simulink model "pv_array"  (R2015a)
settings: Solver=ode45  StartTime=0.0  StopTime=10.0  RelTol=1e-3
libraries: powerlib x4
settings Model: Creator=Limon  LastModifiedBy=Limon

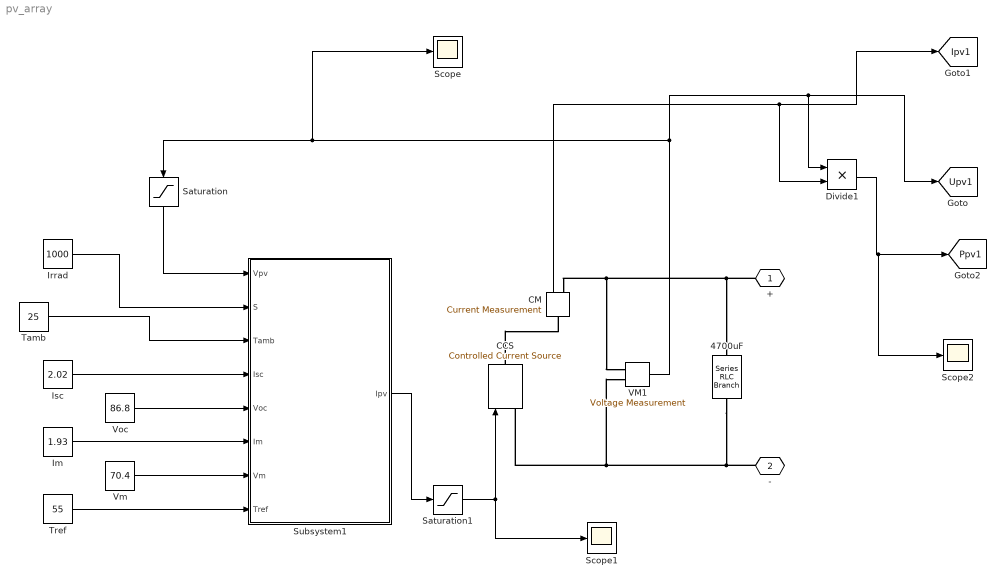
== system pv_array ==
  4700uF : powerlib/Elements/Series RLC Branch  LConnTagsString=__new0  RConnTagsString=__new0  BranchType=C  Resistance=1  Inductance=5e-03  SetiL0=off  InitialCurrent=0  Capacitance=4700e-6  Setx0=off  InitialVoltage=0  Measurements=None
  CCS : powerlib/Electrical Sources/Controlled Current Source  Initialize=on  Source_Type=AC  Amplitude=0  Phase=0  Frequency=0  Measurements=None
  CM : powerlib/Measurements/Current Measurement  PhasorSimulation=off  OutputType=Complex  PSBequivalent=0
  Divide1 : Product  Inputs=**
  Im : Constant  Value=1.93
  "Irrad " : Constant  Value=1000
  Isc : Constant  Value=2.02
  Saturation : Saturate  UpperLimit=100  LowerLimit=0
  Saturation1 : Saturate  UpperLimit=4  LowerLimit=0
  Scope : Scope
  Scope1 : Scope
  Scope2 : Scope
      settings: SaveName=ScopeData2
  Subsystem1 : Subsystem
  "Tamb " : Constant  Value=25
  Tref : Constant  Value=55
  VM1 : powerlib/Measurements/Voltage Measurement  PhasorSimulation=off  OutputType=Complex  PSBequivalent=0
  Vm : Constant  Value=70.4
  Voc : Constant  Value=86.8
  + : PMIOPort  Tag=PMCPort  Port=1  Side=Left
  - : PMIOPort  Tag=PMCPort  Port=2  Side=Right
  tag scope: Ipv1=global, Ppv1=global, Upv1=global
  wires:
  Saturation1/1 -> CCS/1, Scope1/1
  CM/1 -> Divide1/2, [Ipv1]
  Divide1/1 -> Scope2/1, [Ppv1]
  Subsystem1/1(Ipv) -> Saturation1/1
  Tref/1 -> Subsystem1/8(Tref)
  VM1/1 -> Divide1/1, [Upv1], Scope/1, Saturation/1
  Saturation/1 -> Subsystem1/1(Vpv)
  Vm/1 -> Subsystem1/7(Vm)
  Voc/1 -> Subsystem1/5(Voc)
  Im/1 -> Subsystem1/6(Im)
  Isc/1 -> Subsystem1/4(Isc)
  "Tamb "/1 -> Subsystem1/3(Tamb)
  "Irrad "/1 -> Subsystem1/2(S)
  connections:
  -/RConn1 -- 4700uF/RConn1 -- VM1/LConn2 -- CCS/LConn1
  +/RConn1 -- 4700uF/LConn1 -- VM1/LConn1 -- CM/RConn1
  CCS/RConn1 -- CM/LConn1

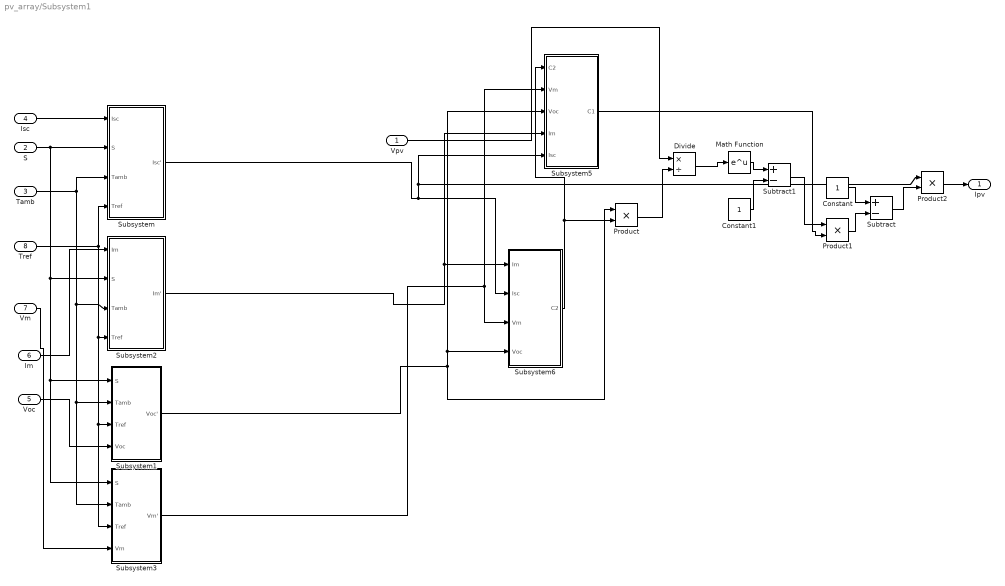
== system pv_array/Subsystem1 ==
  Vpv : Inport
  S : Inport  Port=2
  Tamb : Inport  Port=3
  Isc : Inport  Port=4
  Voc : Inport  Port=5
  Im : Inport  Port=6
  Vm : Inport  Port=7
  Tref : Inport  Port=8
  Constant : Constant
  Constant1 : Constant
  Divide : Product  Inputs=*/
  Math Function : Math  SaturateOnIntegerOverflow=on
  Product : Product  RndMeth=Zero
  Product1 : Product  RndMeth=Zero
  Product2 : Product  RndMeth=Zero
  Subsystem : Subsystem
  Subsystem1 : Subsystem
  Subsystem2 : Subsystem
  Subsystem3 : Subsystem
  Subsystem5 : Subsystem
  Subsystem6 : Subsystem
  Subtract : Sum  Inputs=+-
  Subtract1 : Sum  Inputs=+-
  Ipv : Outport
  wires:
  Vm/1 -> Subsystem3/4(Vm)
  Voc/1 -> Subsystem1/4(Voc)
  Im/1 -> Subsystem2/1(Im)
  Tref/1 -> Subsystem/4(Tref), Subsystem2/4(Tref), Subsystem3/3(Tref), Subsystem1/3(Tref)
  Tamb/1 -> Subsystem/3(Tamb), Subsystem2/3(Tamb), Subsystem3/2(Tamb), Subsystem1/2(Tamb)
  S/1 -> Subsystem/2(S), Subsystem2/2(S), Subsystem3/1(S), Subsystem1/1(S)
  Isc/1 -> Subsystem/1(Isc)
  Subsystem5/1(C1) -> Product1/2
  Vpv/1 -> Divide/1
  Subsystem6/1(C2) -> Product/2, Subsystem5/1(C2)
  Subsystem3/1(Vm') -> Subsystem6/3(Vm), Subsystem5/2(Vm)
  Subsystem1/1(Voc') -> Subsystem6/4(Voc), Subsystem5/3(Voc), Product/1
  Subsystem/1(Isc') -> Subsystem5/5(Isc), Product2/1, Subsystem6/2(Isc)
  Subsystem2/1(Im') -> Subsystem5/4(Im), Subsystem6/1(Im)
  Subtract1/1 -> Product1/1
  Constant1/1 -> Subtract1/2
  Math Function/1 -> Subtract1/1
  Divide/1 -> Math Function/1
  Product2/1 -> Ipv/1
  Subtract/1 -> Product2/2
  Product1/1 -> Subtract/2
  Constant/1 -> Subtract/1
  Product/1 -> Divide/2

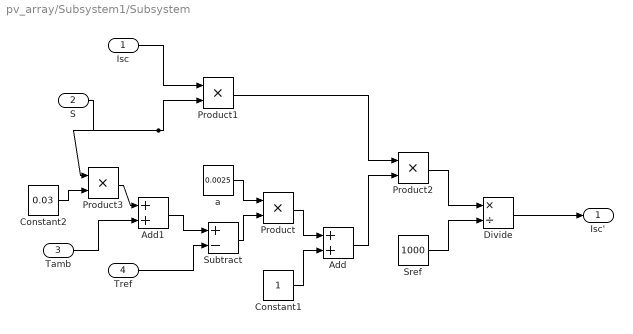
== system pv_array/Subsystem1/Subsystem ==
  Isc : Inport
  S : Inport  Port=2
  Tamb : Inport  Port=3
  Tref : Inport  Port=4
  Add : Sum
  Add1 : Sum
  Constant1 : Constant
  Constant2 : Constant  Value=0.03
  Divide : Product  Inputs=*/
  Product{,1..3} (4 alike) : Product  RndMeth=Zero
  Sref : Constant  Value=1000
  Subtract : Sum  Inputs=+-
  a : Constant  Value=0.0025
  Isc' : Outport
  wires:
  Add1/1 -> Subtract/1
  Tamb/1 -> Add1/2
  Product3/1 -> Add1/1
  Constant2/1 -> Product3/2
  Tref/1 -> Subtract/2
  Divide/1 -> Isc'/1
  Sref/1 -> Divide/2
  Product2/1 -> Divide/1
  Add/1 -> Product2/2
  Product1/1 -> Product2/1
  S/1 -> Product3/1, Product1/2
  Isc/1 -> Product1/1
  Product/1 -> Add/1
  Constant1/1 -> Add/2
  a/1 -> Product/1
  Subtract/1 -> Product/2

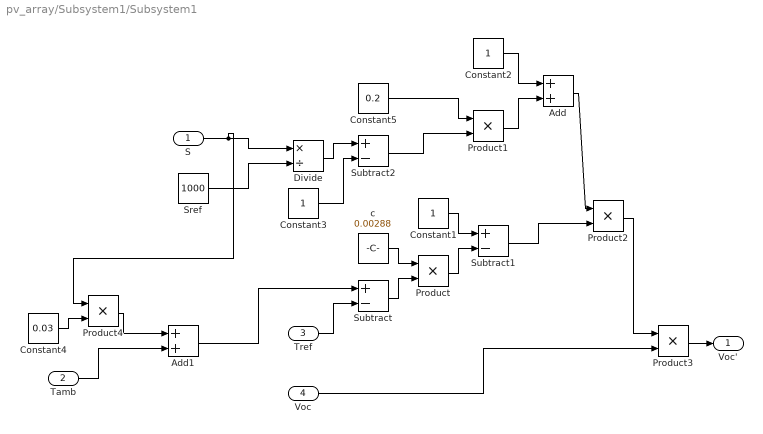
== system pv_array/Subsystem1/Subsystem1 ==
  S : Inport
  Tamb : Inport  Port=2
  Tref : Inport  Port=3
  Voc : Inport  Port=4
  Add : Sum
  Add1 : Sum
  Constant1 : Constant
  Constant2 : Constant
  Constant3 : Constant
  Constant4 : Constant  Value=0.03
  Constant5 : Constant  Value=0.2
  Divide : Product  Inputs=*/
  Product{,1..4} (5 alike) : Product  RndMeth=Zero
  Sref : Constant  Value=1000
  Subtract : Sum  Inputs=+-
  Subtract1 : Sum  Inputs=+-
  Subtract2 : Sum  Inputs=+-
  c : Constant  Value=0.00288
  Voc' : Outport
  wires:
  Constant5/1 -> Product1/1
  Add1/1 -> Subtract/1
  Tamb/1 -> Add1/2
  Product4/1 -> Add1/1
  Constant4/1 -> Product4/2
  Constant3/1 -> Subtract2/2
  Divide/1 -> Subtract2/1
  Sref/1 -> Divide/2
  S/1 -> Product4/1, Divide/1
  Product3/1 -> Voc'/1
  Voc/1 -> Product3/2
  Product2/1 -> Product3/1
  Add/1 -> Product2/1
  Subtract1/1 -> Product2/2
  Product1/1 -> Add/2
  Constant2/1 -> Add/1
  Subtract2/1 -> Product1/2
  Product/1 -> Subtract1/2
  Constant1/1 -> Subtract1/1
  Subtract/1 -> Product/2
  c/1 -> Product/1
  Tref/1 -> Subtract/2

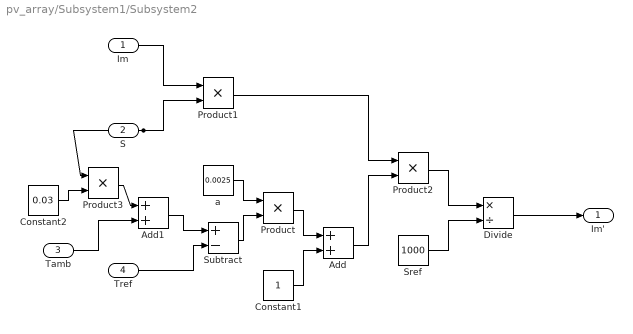
== system pv_array/Subsystem1/Subsystem2 ==
  Im : Inport
  S : Inport  Port=2
  Tamb : Inport  Port=3
  Tref : Inport  Port=4
  Add : Sum
  Add1 : Sum
  Constant1 : Constant
  Constant2 : Constant  Value=0.03
  Divide : Product  Inputs=*/
  Product{,1..3} (4 alike) : Product  RndMeth=Zero
  Sref : Constant  Value=1000
  Subtract : Sum  Inputs=+-
  a : Constant  Value=0.0025
  Im' : Outport
  wires:
  Add1/1 -> Subtract/1
  Tamb/1 -> Add1/2
  Product3/1 -> Add1/1
  Constant2/1 -> Product3/2
  Tref/1 -> Subtract/2
  Divide/1 -> Im'/1
  Sref/1 -> Divide/2
  Product2/1 -> Divide/1
  Add/1 -> Product2/2
  Product1/1 -> Product2/1
  S/1 -> Product1/2, Product3/1
  Im/1 -> Product1/1
  Product/1 -> Add/1
  Constant1/1 -> Add/2
  a/1 -> Product/1
  Subtract/1 -> Product/2

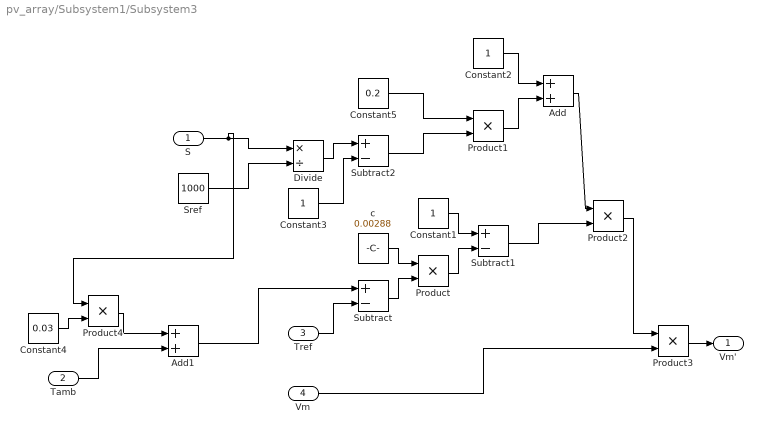
== system pv_array/Subsystem1/Subsystem3 ==
  S : Inport
  Tamb : Inport  Port=2
  Tref : Inport  Port=3
  Vm : Inport  Port=4
  Add : Sum
  Add1 : Sum
  Constant1 : Constant
  Constant2 : Constant
  Constant3 : Constant
  Constant4 : Constant  Value=0.03
  Constant5 : Constant  Value=0.2
  Divide : Product  Inputs=*/
  Product{,1..4} (5 alike) : Product  RndMeth=Zero
  Sref : Constant  Value=1000
  Subtract : Sum  Inputs=+-
  Subtract1 : Sum  Inputs=+-
  Subtract2 : Sum  Inputs=+-
  c : Constant  Value=0.00288
  Vm' : Outport
  wires:
  Constant5/1 -> Product1/1
  Add1/1 -> Subtract/1
  Tamb/1 -> Add1/2
  Product4/1 -> Add1/1
  Constant4/1 -> Product4/2
  Constant3/1 -> Subtract2/2
  Divide/1 -> Subtract2/1
  Sref/1 -> Divide/2
  S/1 -> Product4/1, Divide/1
  Product3/1 -> Vm'/1
  Vm/1 -> Product3/2
  Product2/1 -> Product3/1
  Add/1 -> Product2/1
  Subtract1/1 -> Product2/2
  Product1/1 -> Add/2
  Constant2/1 -> Add/1
  Subtract2/1 -> Product1/2
  Product/1 -> Subtract1/2
  Constant1/1 -> Subtract1/1
  Subtract/1 -> Product/2
  c/1 -> Product/1
  Tref/1 -> Subtract/2

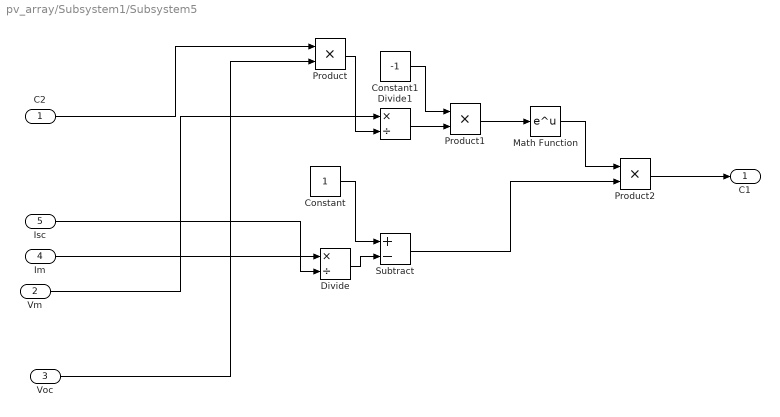
== system pv_array/Subsystem1/Subsystem5 ==
  C2 : Inport
  Vm : Inport  Port=2
  Voc : Inport  Port=3
  Im : Inport  Port=4
  Isc : Inport  Port=5
  Constant : Constant
  Constant1 : Constant  Value=-1
  Divide : Product  Inputs=*/
  Divide1 : Product  Inputs=*/
  Math Function : Math  SaturateOnIntegerOverflow=on
  Product : Product  RndMeth=Zero
  Product1 : Product  RndMeth=Zero
  Product2 : Product  RndMeth=Zero
  Subtract : Sum  Inputs=+-
  C1 : Outport
  wires:
  Divide/1 -> Subtract/2
  Constant/1 -> Subtract/1
  Isc/1 -> Divide/2
  Im/1 -> Divide/1
  C2/1 -> Product/1
  Voc/1 -> Product/2
  Vm/1 -> Divide1/1
  Product2/1 -> C1/1
  Subtract/1 -> Product2/2
  Math Function/1 -> Product2/1
  Product1/1 -> Math Function/1
  Constant1/1 -> Product1/1
  Divide1/1 -> Product1/2
  Product/1 -> Divide1/2

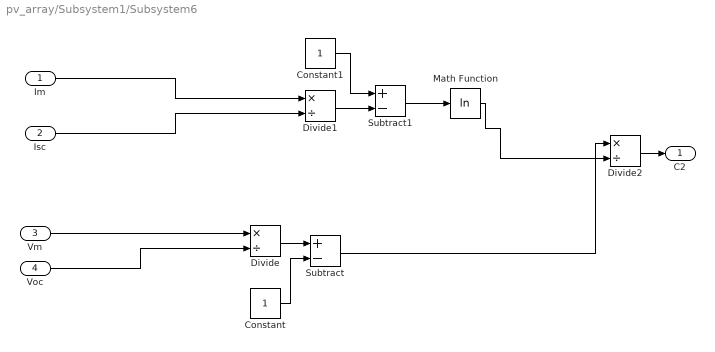
== system pv_array/Subsystem1/Subsystem6 ==
  Im : Inport
  Isc : Inport  Port=2
  Vm : Inport  Port=3
  Voc : Inport  Port=4
  Constant : Constant
  Constant1 : Constant
  Divide : Product  Inputs=*/
  Divide1 : Product  Inputs=*/
  Divide2 : Product  Inputs=*/
  Math Function : Math  Operator=log  SaturateOnIntegerOverflow=on
  Subtract : Sum  Inputs=+-
  Subtract1 : Sum  Inputs=+-
  C2 : Outport
  wires:
  Math Function/1 -> Divide2/2
  Subtract/1 -> Divide2/1
  Subtract1/1 -> Math Function/1
  Isc/1 -> Divide1/2
  Im/1 -> Divide1/1
  Voc/1 -> Divide/2
  Vm/1 -> Divide/1
  Divide2/1 -> C2/1
  Divide1/1 -> Subtract1/2
  Constant1/1 -> Subtract1/1
  Constant/1 -> Subtract/2
  Divide/1 -> Subtract/1
